simulink model "shape_delayNonideal_peakDet_oneShot_atten"  (R2020b)
settings: Solver=VariableStepAuto  StartTime=0.0  StopTime=10.0  RelTol=1e-3
values from neighbouring files (symbols this model uses):
  v_LED = .02    (= 0.02)    [zz_cfd.m]
undefined symbols (not defined in the file or in its folder): f_attenuation
libraries: simulink x4, eeGeneralControl x2
settings Model: Creator=lydialee  LastModifiedBy=lydialee

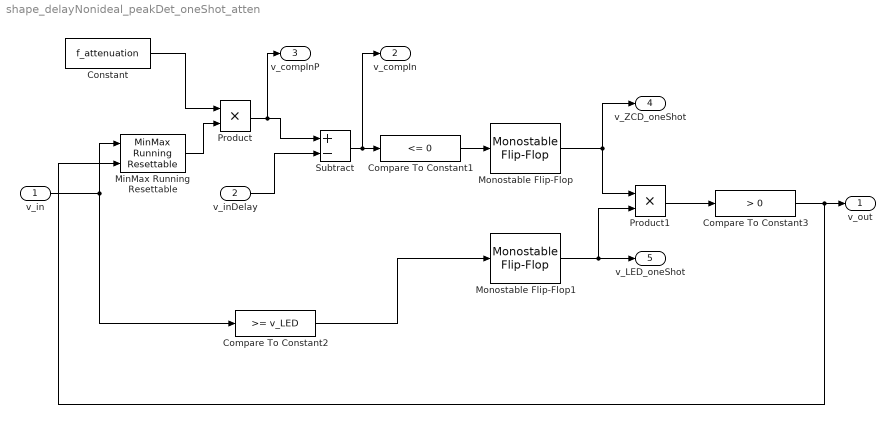
== system shape_delayNonideal_peakDet_oneShot_atten ==
  v_in : Inport
  v_inDelay : Inport  Port=2
  Compare To Constant1 : simulink/Logic and Bit Operations/Compare To Constant  relop=<=  const=0  OutDataTypeStr=boolean
  Compare To Constant2 : simulink/Logic and Bit Operations/Compare To Constant  relop=>=  const=v_LED  OutDataTypeStr=boolean
  Compare To Constant3 : simulink/Logic and Bit Operations/Compare To Constant  relop=>  const=0  OutDataTypeStr=boolean
  Constant : Constant  Value=f_attenuation
  MinMax Running Resettable : simulink/Math Operations/MinMax Running Resettable  Function=max  vinit=0.0
  Monostable Flip-Flop : eeGeneralControl/Monostable Flip-Flop  VariantControl=Variant1  LabelModeActiveChoice=Continuous  ChangeType=Rising edge  x0=0  Td=10e-9  Ts=0
      settings: SourceProductBaseCode=PS
  Monostable Flip-Flop1 : eeGeneralControl/Monostable Flip-Flop  VariantControl=Variant1  LabelModeActiveChoice=Continuous  ChangeType=Rising edge  x0=0  Td=10e-9  Ts=0
      settings: SourceProductBaseCode=PS
  Product : Product
  Product1 : Product
  Subtract : Sum  Inputs=+-
  v_out : Outport  VectorParamsAs1DForOutWhenUnconnected=off
  v_compIn : Outport  Port=2  VectorParamsAs1DForOutWhenUnconnected=off
  v_compInP : Outport  Port=3  VectorParamsAs1DForOutWhenUnconnected=off
  v_ZCD_oneShot : Outport  Port=4  VectorParamsAs1DForOutWhenUnconnected=off
  v_LED_oneShot : Outport  Port=5  VectorParamsAs1DForOutWhenUnconnected=off
  wires:
  Product/1 -> v_compInP/1, Subtract/1
  Constant/1 -> Product/1
  Subtract/1 -> v_compIn/1, Compare To Constant1/1
  v_in/1 -> MinMax Running Resettable/1, Compare To Constant2/1
  v_inDelay/1 -> Subtract/2
  Compare To Constant1/1 -> Monostable Flip-Flop/1
  Compare To Constant2/1 -> Monostable Flip-Flop1/1
  Monostable Flip-Flop/1 -> Product1/1, v_ZCD_oneShot/1
  Monostable Flip-Flop1/1 -> v_LED_oneShot/1, Product1/2
  MinMax Running Resettable/1 -> Product/2
  Product1/1 -> Compare To Constant3/1
  Compare To Constant3/1 -> MinMax Running Resettable/2, v_out/1
